simulink model "notLinModel_S_cc"  (R2022a)
settings: Solver=ode45  StartTime=0.0  StopTime=2  MaxStep=0.001  RelTol=1e-9
values from neighbouring files (symbols this model uses):
  c = 0.75    [Operation_.m]
  C_magnetic = 3.73e-6    (= 3.73e-06)    [Operation_.m]
  gap = 3E-4    (= 0.0003)    [Operation_.m]
  k = 345.0    (= 345)    [Operation_.m]
  Kr = lqr(A,B,Q,R)    [Operation_.m]
  mass = k/(4.5*2*pi)^2    (= 0.431553189588)    [Operation_.m]
settings Model: Creator=danli  LastModifiedBy=danli
settings SolverCC: AlgebraicLoopSolver=TrustRegion
settings DebuggingCC: UnconnectedInputMsg=warning  UnconnectedOutputMsg=warning  UnconnectedLineMsg=warning  SFMachineParentedDataDiag=warning
settings RTWCC: DLArmComputeVersion=19.05

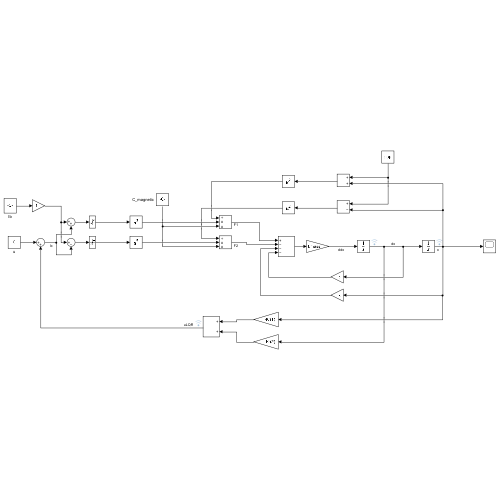
[thumbnail: Simulink's stored preview of the top-level diagram]
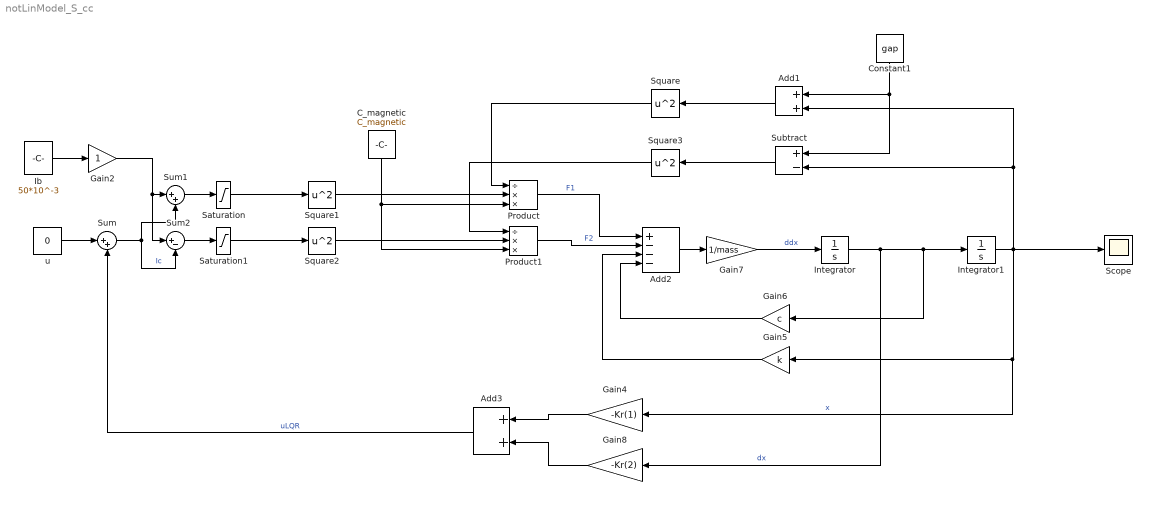
== system notLinModel_S_cc ==
  Add1 : Sum
  Add2 : Sum  Inputs=+---
  Add3 : Sum
  C_magnetic : Constant  Value=C_magnetic
  Constant1 : Constant  Value=gap
  Gain2 : Gain
  Gain4 : Gain  Gain=-Kr(1)
  Gain5 : Gain  Gain=k
  Gain6 : Gain  Gain=c
  Gain7 : Gain  Gain=1/mass
  Gain8 : Gain  Gain=-Kr(2)
  Ib : Constant  Value=50*10^-3
  Integrator : Integrator
  Integrator1 : Integrator  InitialCondition=50*10^-6
  Product : Product  Inputs=/**
  Product1 : Product  Inputs=/**
  Saturation : Saturate  UpperLimit=2  LowerLimit=0
  Saturation1 : Saturate  UpperLimit=2  LowerLimit=0
  Scope : Scope
  Square{,1..3} (4 alike) : Math  Operator=square
  Subtract : Sum  Inputs=+-
  Sum : Sum  Inputs=|++
  Sum1 : Sum  Inputs=|++
  Sum2 : Sum  Inputs=|+-
  u : Constant  Value=0
  wires:
  Ib/1 -> Gain2/1
  Sum1/1 -> Saturation/1
  Sum2/1 -> Saturation1/1
  Sum/1 -> Sum1/2, Sum2/2  "Ic"
  Gain2/1 -> Sum2/1, Sum1/1
  Integrator1/1 -> Gain4/1, Gain5/1, Scope/1, Add1/2, Subtract/2  "x"
  Saturation1/1 -> Square2/1
  Saturation/1 -> Square1/1
  Square2/1 -> Product1/2
  Constant1/1 -> Subtract/1, Add1/1
  Square1/1 -> Product/2
  Gain6/1 -> Add2/4
  Integrator/1 -> Gain8/1, Gain6/1, Integrator1/1  "dx"
  Gain5/1 -> Add2/3
  Product1/1 -> Add2/2  "F2"
  Subtract/1 -> Square3/1
  Square/1 -> Product/1
  Add1/1 -> Square/1
  Add2/1 -> Gain7/1
  Product/1 -> Add2/1  "F1"
  Square3/1 -> Product1/1
  C_magnetic/1 -> Product/3, Product1/3
  Gain7/1 -> Integrator/1  "ddx"
  u/1 -> Sum/1
  Gain4/1 -> Add3/1
  Gain8/1 -> Add3/2
  Add3/1 -> Sum/2  "uLQR"
